simulink model "c2_wideband_filter"  (R2020b)
settings: Solver=FixedStepDiscrete  StartTime=0.0  StopTime=stopTime  FixedStep=2.0833333333333333e-05  RelTol=1e-3
values from neighbouring files (symbols this model uses):
  C2coeffs = zeros(5,6)    [C2Coefficients.m]
undefined symbols (not defined in the file or in its folder): cf, norm_gainc2
settings Model: Creator=Ross  LastModifiedBy=conno
settings DataIOCC: SaveOutput=off  SaveTime=off  ReturnWorkspaceOutputs=off
settings OptimizationCC: BlockReduction=off  ConditionallyExecuteInputs=off  DefaultParameterBehavior=Inlined
settings DebuggingCC: ReadBeforeWriteMsg=DisableAll  WriteAfterWriteMsg=DisableAll  WriteAfterReadMsg=DisableAll  AlgebraicLoopMsg=error  MultiTaskDSMMsg=none  SingleTaskRateTransMsg=error  PregeneratedLibrarySubsystemCodeDiagnostic=none  ArithmeticOperatorsInVariantConditions=warning
settings HardwareCC: ProdBitPerPointer=32  ProdBitPerSizeT=32  ProdBitPerPtrDiffT=32  ProdLargestAtomicFloat=None  ProdIntDivRoundTo=Undefined  ProdEndianess=Unspecified  ProdWordSize=32  ProdHWDeviceType=ASIC/FPGA->ASIC/FPGA  TargetBitPerPointer=64  TargetBitPerSizeT=64  TargetBitPerPtrDiffT=64  TargetLongLongMode=on  TargetIntDivRoundTo=Zero  TargetEndianess=LittleEndian  TargetWordSize=64  TargetHWDeviceType=Custom Processor->MATLAB Host Computer  ProdEqTarget=off
settings ModelReferenceCC: UpdateModelReferenceTargets=IfOutOfDate
settings SFSimCC: SFSimEcho=off  SimUseLocalCustomCode=off  CustomCodeUndefinedFunction=UseInterfaceOnly
settings RTWCC: RTWUseLocalCustomCode=off

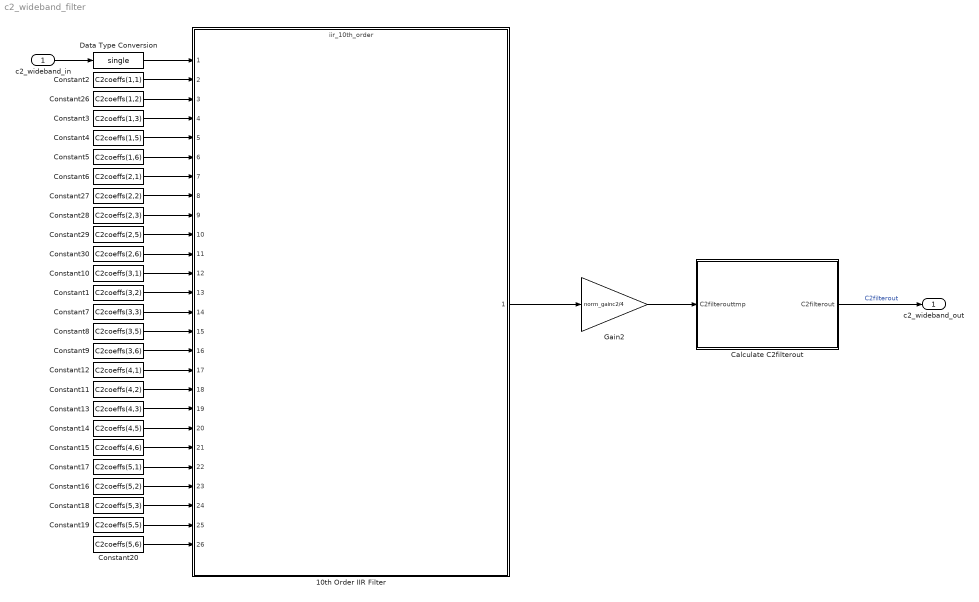
== system c2_wideband_filter ==
  c2_wideband_in : Inport  OutDataTypeStr=single  PortDimensions=1  SampleTime=[2.0833333333333333e-05,0]
  10th Order IIR Filter : ModelReference  ModelNameDialog=iir_10th_order  SimulationMode=Normal  ModelReferenceVersion=1.113
  Calculate C2filterout : Subsystem
  Constant1 : Constant  Value=C2coeffs(3,2)  OutDataTypeStr=single  SampleTime=-1
  Constant10 : Constant  Value=C2coeffs(3,1)  OutDataTypeStr=single  SampleTime=-1
  Constant11 : Constant  Value=C2coeffs(4,2)  OutDataTypeStr=single  SampleTime=-1
  Constant12 : Constant  Value=C2coeffs(4,1)  OutDataTypeStr=single  SampleTime=-1
  Constant13 : Constant  Value=C2coeffs(4,3)  OutDataTypeStr=single  SampleTime=-1
  Constant14 : Constant  Value=C2coeffs(4,5)  OutDataTypeStr=single  SampleTime=-1
  Constant15 : Constant  Value=C2coeffs(4,6)  OutDataTypeStr=single  SampleTime=-1
  Constant16 : Constant  Value=C2coeffs(5,2)  OutDataTypeStr=single  SampleTime=-1
  Constant17 : Constant  Value=C2coeffs(5,1)  OutDataTypeStr=single  SampleTime=-1
  Constant18 : Constant  Value=C2coeffs(5,3)  OutDataTypeStr=single  SampleTime=-1
  Constant19 : Constant  Value=C2coeffs(5,5)  OutDataTypeStr=single  SampleTime=-1
  Constant2 : Constant  Value=C2coeffs(1,1)  OutDataTypeStr=single  SampleTime=-1
  Constant20 : Constant  Value=C2coeffs(5,6)  OutDataTypeStr=single  SampleTime=-1
  Constant26 : Constant  Value=C2coeffs(1,2)  OutDataTypeStr=single  SampleTime=-1
  Constant27 : Constant  Value=C2coeffs(2,2)  OutDataTypeStr=single  SampleTime=-1
  Constant28 : Constant  Value=C2coeffs(2,3)  OutDataTypeStr=single  SampleTime=-1
  Constant29 : Constant  Value=C2coeffs(2,5)  OutDataTypeStr=single  SampleTime=-1
  Constant3 : Constant  Value=C2coeffs(1,3)  OutDataTypeStr=single  SampleTime=-1
  Constant30 : Constant  Value=C2coeffs(2,6)  OutDataTypeStr=single  SampleTime=-1
  Constant4 : Constant  Value=C2coeffs(1,5)  OutDataTypeStr=single  SampleTime=-1
  Constant5 : Constant  Value=C2coeffs(1,6)  OutDataTypeStr=single  SampleTime=-1
  Constant6 : Constant  Value=C2coeffs(2,1)  OutDataTypeStr=single  SampleTime=-1
  Constant7 : Constant  Value=C2coeffs(3,3)  OutDataTypeStr=single  SampleTime=-1
  Constant8 : Constant  Value=C2coeffs(3,5)  OutDataTypeStr=single  SampleTime=-1
  Constant9 : Constant  Value=C2coeffs(3,6)  OutDataTypeStr=single  SampleTime=-1
  Data Type Conversion : DataTypeConversion  OutDataTypeStr=single
  Gain2 : Gain  Gain=norm_gainc2/4
  c2_wideband_out : Outport  OutDataTypeStr=single  PortDimensions=1  SampleTime=[2.0833333333333333e-05,0]  InitialOutput=0  VectorParamsAs1DForOutWhenUnconnected=off
  wires:
  c2_wideband_in/1 -> Data Type Conversion/1
  10th Order IIR Filter/1 -> Gain2/1
  Gain2/1 -> Calculate C2filterout/1(C2filterouttmp)
  Calculate C2filterout/1(C2filterout) -> c2_wideband_out/1  "C2filterout"
  Constant1/1 -> 10th Order IIR Filter/13
  Constant26/1 -> 10th Order IIR Filter/3
  Constant12/1 -> 10th Order IIR Filter/17
  Constant19/1 -> 10th Order IIR Filter/25
  Constant18/1 -> 10th Order IIR Filter/24
  Constant15/1 -> 10th Order IIR Filter/21
  Constant11/1 -> 10th Order IIR Filter/18
  Constant2/1 -> 10th Order IIR Filter/2
  Data Type Conversion/1 -> 10th Order IIR Filter/1
  Constant4/1 -> 10th Order IIR Filter/5
  Constant7/1 -> 10th Order IIR Filter/14
  Constant14/1 -> 10th Order IIR Filter/20
  Constant13/1 -> 10th Order IIR Filter/19
  Constant20/1 -> 10th Order IIR Filter/26
  Constant30/1 -> 10th Order IIR Filter/11
  Constant28/1 -> 10th Order IIR Filter/9
  Constant10/1 -> 10th Order IIR Filter/12
  Constant17/1 -> 10th Order IIR Filter/22
  Constant9/1 -> 10th Order IIR Filter/16
  Constant6/1 -> 10th Order IIR Filter/7
  Constant27/1 -> 10th Order IIR Filter/8
  Constant8/1 -> 10th Order IIR Filter/15
  Constant3/1 -> 10th Order IIR Filter/4
  Constant5/1 -> 10th Order IIR Filter/6
  Constant16/1 -> 10th Order IIR Filter/23
  Constant29/1 -> 10th Order IIR Filter/10

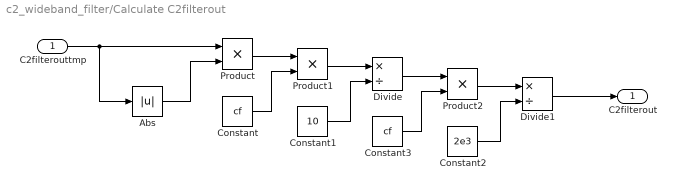
== system c2_wideband_filter/Calculate C2filterout ==
  C2filterouttmp : Inport
  Abs : Abs
  Constant : Constant  Value=cf  OutDataTypeStr=single  SampleTime=-1
  Constant1 : Constant  Value=10  OutDataTypeStr=single  SampleTime=-1
  Constant2 : Constant  Value=2e3  OutDataTypeStr=single  SampleTime=-1
  Constant3 : Constant  Value=cf  OutDataTypeStr=single  SampleTime=-1
  Divide : Product  Inputs=*/  RndMeth=Zero  SaturateOnIntegerOverflow=on
  Divide1 : Product  Inputs=*/  RndMeth=Zero  SaturateOnIntegerOverflow=on
  Product : Product
  Product1 : Product
  Product2 : Product
  C2filterout : Outport  VectorParamsAs1DForOutWhenUnconnected=off
  wires:
  C2filterouttmp/1 -> Product/1, Abs/1
  Abs/1 -> Product/2
  Product/1 -> Product1/1
  Constant/1 -> Product1/2
  Product1/1 -> Divide/1
  Constant1/1 -> Divide/2
  Product2/1 -> Divide1/1
  Constant2/1 -> Divide1/2
  Constant3/1 -> Product2/2
  Divide/1 -> Product2/1
  Divide1/1 -> C2filterout/1
